simulink model "PD_Controller"  (R2025b)
settings: Solver=FixedStepAuto  StartTime=0.0  StopTime=inf  FixedStep=0.002  RelTol=1e-3  EnableMultiTasking=on
undefined symbols (not defined in the file): HIL, qc_get_step_size
libraries: quarc_library x5, simulink x1, simulink_extras x1
settings Model: ExtModeTrigDuration=10000  Creator=henrr  LastModifiedBy=henrr
settings SolverCC: AlgebraicLoopSolver=TrustRegion  PositivePriorityOrder=on
settings DataIOCC: ReturnWorkspaceOutputs=off
settings DebuggingCC: UnconnectedInputMsg=warning  UnconnectedOutputMsg=warning  UnconnectedLineMsg=warning  ArithmeticOperatorsInVariantConditions=warning
settings ModelReferenceCC: EnableRefExpFcnMdlSchedulingChecks=on
settings SFSimCC: SimUseLocalCustomCode=off  CustomCodeUndefinedFunction=UseInterfaceOnly
settings RTWCC: SystemTargetFile=quarc_win64.tlc  TemplateMakefile=quarc_default_tmf  RTWUseLocalCustomCode=off  Toolchain=QUARC win64 | nmake (64-bit Windows)  BuildConfiguration=Faster Runs  GPUComputeCapability=3.5  Description=QUARC Win64 Target Using Toolchain
settings CodeAppCC: StateflowObjectComments=on
settings STFCustomTargetCC: SystemTargetFile=quarc_win64.tlc  TargetLangStandard=C99 (ISO)  UseToolchainInfoCompliant=on
settings GRTTargetCC: ExtMode=on  ExtModeMexFile=quarc_comm  ParMdlRefBuildCompliant=off  CompOptLevelCompliant=off  CombineOutputUpdateFcns=off  MatFileLogging=off  CPPClassGenCompliant=off  GRTInterface=on
settings ConfigComp: CovMetricSettings=dswe

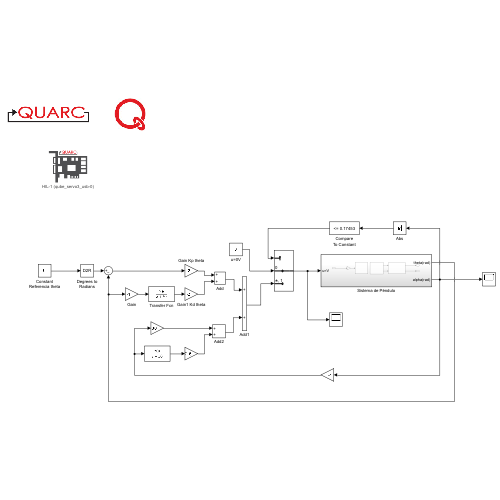
[thumbnail: Simulink's stored preview of the top-level diagram]
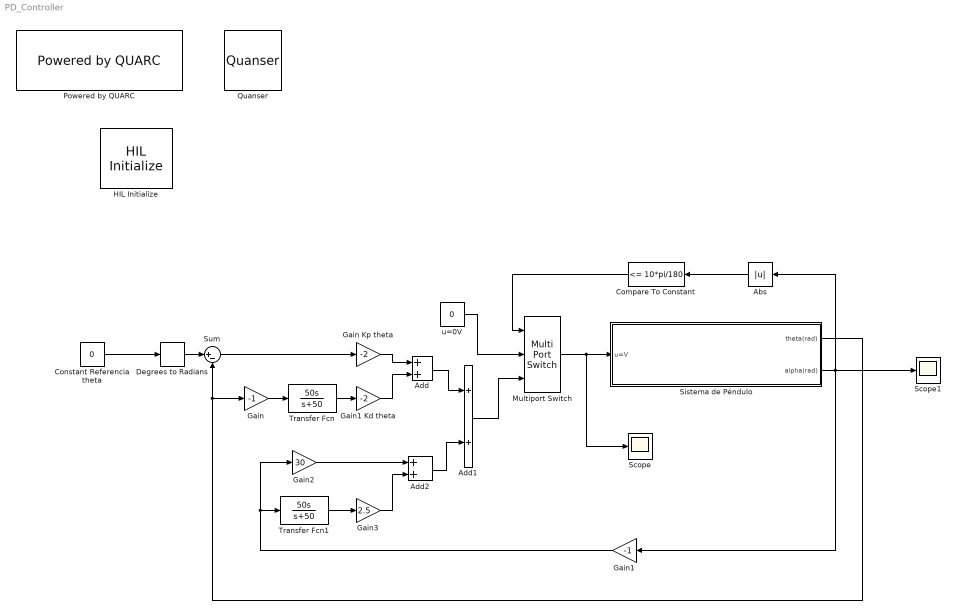
== system PD_Controller ==
  Abs : Abs  SaturateOnIntegerOverflow=off
  Add : Sum
  Add1 : Sum
  Add2 : Sum
  Compare To Constant : simulink/Logic and Bit Operations/Compare To Constant  relop=<=  const=10*pi/180  OutDataTypeStr=boolean
  Constant Referencia theta : Constant  Value=0
  Degrees to Radians : simulink_extras/Transformations/Degrees to Radians
  Gain : Gain  Gain=-1
  Gain Kp theta : Gain  Gain=-2
  Gain1 : Gain  Gain=-1
  Gain1 Kd theta : Gain  Gain=-2
  Gain2 : Gain  Gain=30
  Gain3 : Gain  Gain=2.5
  HIL Initialize : quarc_library/Data Acquisition/Generic/Configuration/HIL Initialize  object_name=HIL-1  board_type=qube_servo3_usb  board_number=0  board_options=deadband_compensation=0.3;pwm_en=0;enc0_velocity=3.0;enc1_velocity=3.0;min_diode_compensation=0.3;max_diode_compensation=1.5  exclusive=off  active=on  hardware_clocks=[0]  clock_modes=[]  initial_clock_frequencies=[]  set_clock_params_at_start=off  set_clock_params_at_switch_in=off  set_clock_frequencies_at_start=off  set_clock_frequencies_at_switch_in=off  analog_input_channels=[0]  analog_input_configurations=[]  analog_input_maximums=3  analog_input_minimums=-3  set_analog_input_params_at_start=off  set_analog_input_params_at_switch_in=off  analog_output_channels=[0]  analog_output_maximums=15  analog_output_minimums=-15  initial_analog_outputs=[0]  final_analog_outputs=[0]  watchdog_analog_outputs=0  set_analog_output_params_at_start=off  set_analog_output_params_at_switch_in=off  set_analog_outputs_at_start=on  set_analog_outputs_at_switch_in=off  set_analog_outputs_at_terminate=on  set_analog_outputs_at_switch_out=off  set_analog_outputs_on_watchdog=on  digital_input_channels=[]  digital_output_channels=[0]  digital_output_configuration=[]  initial_digital_outputs=[1]  final_digital_outputs=[0]  watchdog_digital_outputs=[0]  set_digital_output_params_at_start=off  set_digital_output_params_at_switch_in=off  set_digital_outputs_at_start=on  set_digital_outputs_at_switch_in=off  set_digital_outputs_at_terminate=on  set_digital_outputs_at_switch_out=off  set_digital_outputs_on_watchdog=on  encoder_channels=[0:1]  quadrature=[4]  encoder_filter_frequency=[]  initial_encoder_counts=[0]  set_encoder_params_at_start=off  set_encoder_params_at_switch_in=off  set_encoder_counts_at_start=on  set_encoder_counts_at_switch_in=off  pwm_channels=[]  pwm_modes=[0]  pwm_frequency=23195  pwm_configuration=[1]  pwm_alignment=[0]  pwm_polarity=[1]  pwm_leading_deadband=[0]  pwm_trailing_deadband=[0]  initial_pwm_outputs=[0]  final_pwm_outputs=[0]  watchdog_pwm_outputs=[]  set_pwm_params_at_start=off  set_pwm_params_at_switch_in=off  set_pwm_outputs_at_start=off  set_pwm_outputs_at_switch_in=off  set_pwm_outputs_at_terminate=off  set_pwm_outputs_at_switch_out=off  set_pwm_outputs_on_watchdog=off  other_output_channels=[11000:11002]  initial_other_outputs=[0 1 0]  final_other_outputs=[1 0 0]  watchdog_other_outputs=[0 0 1]  set_other_outputs_at_start=on  set_other_outputs_at_switch_in=off  set_other_outputs_at_terminate=on  set_other_outputs_at_switch_out=off  set_other_outputs_on_watchdog=on
  Multiport Switch : MultiPortSwitch  DataPortOrder=Zero-based contiguous  Inputs=2  zeroidx=on  SaturateOnIntegerOverflow=off  InputSameDT=off
  Powered by QUARC : quarc_library/Logos/Powered by QUARC
  Quanser : quarc_library/Logos/Quanser
  Scope : Scope
      settings: ActiveDisplayYMinimum=-1  ActiveDisplayYMaximum=1
  Scope1 : Scope
      settings: ActiveDisplayYMinimum=3.1020926483017375  ActiveDisplayYMaximum=3.1289373120897368
  Sistema de Péndulo : Subsystem
  Sum : Sum  Inputs=|+-
  Transfer Fcn : TransferFcn  Numerator=[50 0]  Denominator=[1 50]
  Transfer Fcn1 : TransferFcn  Numerator=[50 0]  Denominator=[1 50]
  u=0V : Constant  Value=0
  wires:
  Sistema de Péndulo/2(alpha(rad)) -> Scope1/1, Gain1/1, Abs/1
  Abs/1 -> Compare To Constant/1
  Compare To Constant/1 -> Multiport Switch/1
  Multiport Switch/1 -> Scope/1, Sistema de Péndulo/1(u=V)
  u=0V/1 -> Multiport Switch/2
  Sistema de Péndulo/1(theta(rad)) -> Sum/2, Gain/1
  Degrees to Radians/1 -> Sum/1
  Constant Referencia theta/1 -> Degrees to Radians/1
  Sum/1 -> Gain Kp theta/1
  Gain Kp theta/1 -> Add/1
  Gain/1 -> Transfer Fcn/1
  Transfer Fcn/1 -> Gain1 Kd theta/1
  Gain1 Kd theta/1 -> Add/2
  Add/1 -> Add1/1
  Gain1/1 -> Transfer Fcn1/1, Gain2/1
  Transfer Fcn1/1 -> Gain3/1
  Gain3/1 -> Add2/2
  Gain2/1 -> Add2/1
  Add2/1 -> Add1/2
  Add1/1 -> Multiport Switch/3

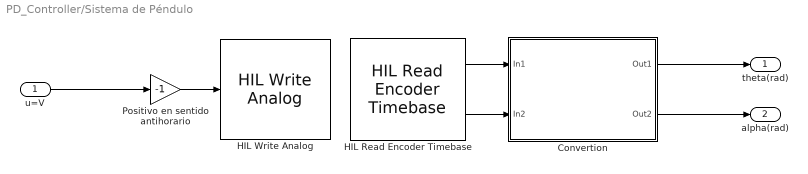
== system PD_Controller/Sistema de Péndulo ==
  u=V : Inport
  Convertion : Subsystem
  HIL Read Encoder Timebase : quarc_library/Data Acquisition/Generic/Timebases/HIL Read Encoder Timebase  object_name=HIL-1  clock=0  channels=[0:1]  active=on  vector_output=off  data_type_mode=Inherit via back propagation  data_type=double  overflow_mode=Error on overflow  samples_in_buffer=max(ceil(1/qc_get_step_size), 1)
  HIL Write Analog : quarc_library/Data Acquisition/Generic/Immediate I//O/HIL Write Analog  object_name=HIL-1  channels=0  sample_time=-1  active=off  vector_input=off
  "Positivo en sentido antihorario " : Gain  Gain=-1
  theta(rad) : Outport
  alpha(rad) : Outport  Port=2
  wires:
  HIL Read Encoder Timebase/1 -> Convertion/1(In1)
  "Positivo en sentido antihorario "/1 -> HIL Write Analog/1
  HIL Read Encoder Timebase/2 -> Convertion/2(In2)
  Convertion/2(Out2) -> alpha(rad)/1
  u=V/1 -> "Positivo en sentido antihorario "/1
  Convertion/1(Out1) -> theta(rad)/1

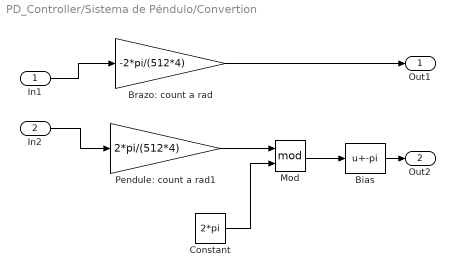
== system PD_Controller/Sistema de Péndulo/Convertion ==
  In1 : Inport
  In2 : Inport  Port=2
  Bias : Bias  Bias=-pi  SaturateOnIntegerOverflow=off
  Brazo: count a rad : Gain  Gain=-2*pi/(512*4)
  Constant : Constant  Value=2*pi
  Mod : Math  Operator=mod
  Pendule: count a rad1 : Gain  Gain=2*pi/(512*4)
  Out1 : Outport
  Out2 : Outport  Port=2
  wires:
  In1/1 -> Brazo: count a rad/1
  In2/1 -> Pendule: count a rad1/1
  Constant/1 -> Mod/2
  Brazo: count a rad/1 -> Out1/1
  Mod/1 -> Bias/1
  Pendule: count a rad1/1 -> Mod/1
  Bias/1 -> Out2/1
